simulink model "simulink_laba_2"  (R2023b)
settings: Solver=VariableStepAuto  StartTime=0.0  StopTime=10.0  RelTol=1e-3
settings Model: Creator=dimon  LastModifiedBy=dimon

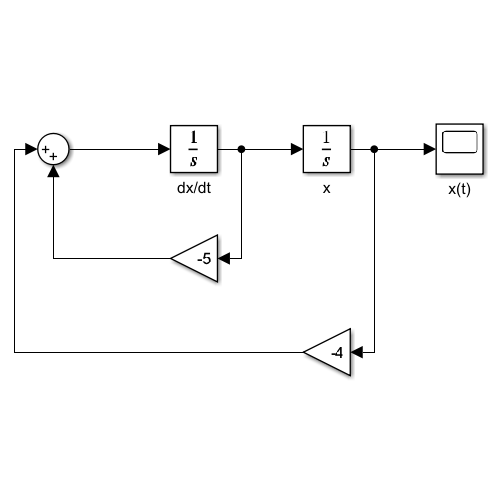
[thumbnail: Simulink's stored preview of the top-level diagram]
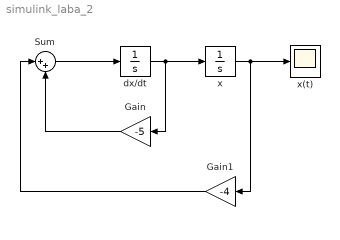
== system simulink_laba_2 ==
  Gain : Gain  Gain=-5
  Gain1 : Gain  Gain=-4
  Sum : Sum  Inputs=|++
  dx/dt : Integrator  InitialCondition=1
  x : Integrator
  x(t) : Scope
  wires:
  Sum/1 -> dx/dt/1
  dx/dt/1 -> Gain/1, x/1
  x/1 -> Gain1/1, x(t)/1
  Gain/1 -> Sum/2
  Gain1/1 -> Sum/1
